simulink model "QPSK_BladeRF_tx"  (R2023a)
settings: Solver=FixedStepDiscrete  StartTime=0.0  StopTime=inf  RelTol=1e-3
undefined symbols (not defined in the file or in its folder): sdrqpsktx
libraries: dspsigops x2, commsequence2 x2, dspsrcs4 x2, commdigbbndpm3 x2, commfilt2 x2
settings Model: SimulationMode=accelerator  Creator=memre  LastModifiedBy=memre
settings DebuggingCC: ParameterPrecisionLossMsg=none
settings HardwareCC: ProdBitPerLong=64  ProdHWDeviceType=Intel->x86-64 (Linux 64)
settings RTWCC: Description=Simulink Desktop Real-Time  SystemTargetFile=sldrt.tlc  TemplateMakefile=sldrt.tmf  RTWCompilerOptimization=on
settings CodeAppCC: MaxIdLength=95
settings SimulinkDesktopRealTimeCC: TargetLibSuffix=_sldrt.a  TargetPreCompLibLocation=C:\Program Files\MATLAB\R2023a\toolbox\sldrt\lib\win64

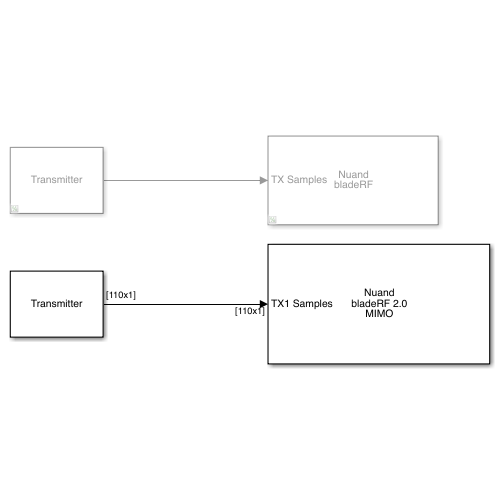
[thumbnail: Simulink's stored preview of the top-level diagram]
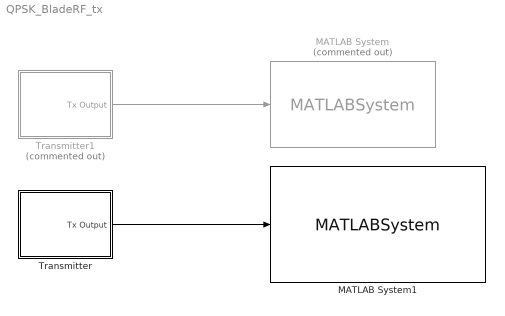
== system QPSK_BladeRF_tx ==
  MATLAB System : MATLABSystem  Commented=on  System=bladeRF_Simulink  device_string=*:instance=1  loopback_mode=None  xb200=off  SimulateUsing=Interpreted execution  enable_rx=off  enable_overrun=off  rx_frequency=sdrqpsktx.BladeRF_Frequency  rx_samplerate=sdrqpsktx.BladeRF_SampleRate  rx_bandwidth=1.5  rx_gain=sdrqpsktx.BladeRF_Gain_Rx  enable_rx_biastee=off  rx_agc=SLOW  rx_num_buffers=sdrqpsktx.BladeRF.stream.n_buffers  rx_num_transfers=sdrqpsktx.BladeRF.stream.n_transfers  rx_buf_size=sdrqpsktx.BladeRF.stream.buffer_size  rx_timeout_ms=sdrqpsktx.BladeRF.stream.timeout  rx_step_size=sdrqpsktx.BladeRF_FrameLength  enable_tx=on  enable_underrun=off  tx_frequency=sdrqpsktx.BladeRF_Frequency  tx_samplerate=sdrqpsktx.BladeRF_SampleRate  tx_bandwidth=1.5  tx_gain=sdrqpsktx.BladeRF_Gain_Tx  enable_tx_biastee=off  tx_num_buffers=sdrqpsktx.BladeRF.stream.n_buffers  tx_num_transfers=sdrqpsktx.BladeRF.stream.n_transfers  tx_buf_size=sdrqpsktx.BladeRF.stream.buffer_size  tx_timeout_ms=sdrqpsktx.BladeRF.stream.timeout  tx_step_size=sdrqpsktx.BladeRF_FrameLength  verbosity=Info
      mask Type: bladeRF_Simulink
      mask Display:
      | disp(['Nuand' char(10) 'bladeRF']);
      | port_label('input',1,'TX Samples');
  MATLAB System1 : MATLABSystem  System=bladeRF_MIMO_Simulink  device_string=*:instance=1  loopback_mode=None  xb200=off  SimulateUsing=Interpreted execution  enable_rx=off  enable_overrun=off  rx_frequency=sdrqpsktx.BladeRF_Frequency  rx_samplerate=sdrqpsktx.BladeRF_SampleRate  rx_bandwidth=1.5  rx_gain=sdrqpsktx.BladeRF_Gain_Rx  enable_rx_biastee=off  rx_agc=SLOW  rx_num_buffers=sdrqpsktx.BladeRF.stream.n_buffers  rx_num_transfers=sdrqpsktx.BladeRF.stream.n_transfers  rx_buf_size=sdrqpsktx.BladeRF.stream.buffer_size  rx_timeout_ms=sdrqpsktx.BladeRF.stream.timeout  rx_step_size=sdrqpsktx.BladeRF_FrameLength  enable_rx2=off  rx2_frequency=sdrqpsktx.BladeRF_Frequency  rx2_samplerate=sdrqpsktx.BladeRF_SampleRate  rx2_bandwidth=1.5  rx2_gain=sdrqpsktx.BladeRF_Gain_Rx  enable_rx2_biastee=off  rx2_agc=SLOW  enable_tx=on  enable_underrun=off  tx_frequency=sdrqpsktx.BladeRF_Frequency  tx_samplerate=sdrqpsktx.BladeRF_SampleRate  tx_bandwidth=1.5  tx_gain=sdrqpsktx.BladeRF_Gain_Tx  enable_tx_biastee=off  tx_num_buffers=sdrqpsktx.BladeRF.stream.n_buffers  tx_num_transfers=sdrqpsktx.BladeRF.stream.n_transfers  tx_buf_size=sdrqpsktx.BladeRF.stream.buffer_size  tx_timeout_ms=sdrqpsktx.BladeRF.stream.timeout  tx_step_size=sdrqpsktx.BladeRF_FrameLength  enable_tx2=off  tx2_frequency=sdrqpsktx.BladeRF_Frequency  tx2_samplerate=sdrqpsktx.BladeRF_SampleRate  tx2_bandwidth=1.5  tx2_gain=sdrqpsktx.BladeRF_Gain_Tx  enable_tx2_biastee=off  verbosity=Info
      mask Type: bladeRF_MIMO_Simulink
      mask Display:
      | disp(['Nuand' char(10) 'bladeRF 2.0' char(10) 'MIMO']);
      | port_label('input',1,'TX1 Samples');
  Transmitter : Subsystem
      mask Display: disp('Transmitter')
  Transmitter1 : Subsystem  Commented=on
      mask Display: disp('Transmitter')
  wires:
  Transmitter/1(Tx Output) -> MATLAB System1/1
  Transmitter1/1(Tx Output) -> MATLAB System/1

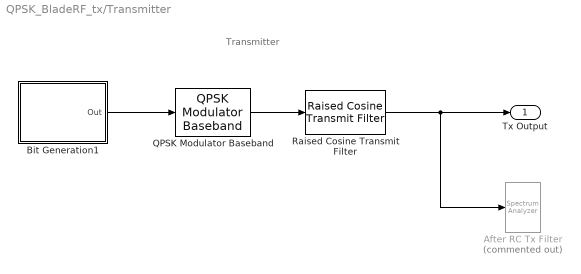
== system QPSK_BladeRF_tx/Transmitter ==
  note: Transmitter
  After RC Tx Filter : SpectrumAnalyzer  Commented=on  ScopeFrameLocation=window  Method=Welch  SampleRate=200000  Span=200000  StartFrequency=-100000  StopFrequency=100000  RBWSource=Property  RBW=750  FFTLength=128  AveragingMethod=Running  SpectralAverages=2  SpectrumUnits=dBW  YLabel=Spectrum after Raised-Cosine Tx Filter  YLimits=[-114.15736879359562 -6.4493918406395565]
      settings: OpenAtSimulationStart=off
  Bit Generation1 : Subsystem
      mask Display: disp('Bits Generation')
  QPSK Modulator Baseband : commdigbbndpm3/QPSK Modulator Baseband  InType=Bit  Enc=Gray  Ph=pi/4  outDtype=double  outWordLen=16  outUDDataType=sfix(16)  outFracLenMode=Best precision  outFracLen=15  outDataTypeStr=double  outLastDataTypeStr=double
  Raised Cosine Transmit Filter : commfilt2/Raised Cosine Transmit Filter  filtType=Square root  R=sdrqpsktx.RolloffFactor  filtSpan=sdrqpsktx.RaisedCosineFilterSpan  N=sdrqpsktx.Interpolation  filterGain=1  InputProcessing=Columns as channels (frame based)  RateOptions=Enforce single-rate processing  framing=Mute  checkCoeff=off  variableName=rcTxFilt1  checkGain=Normalized  sampMode=Mute  saveAsFlag=0  currentFiltSpan=10  D=5  launchFVT=on  roundingMode=Floor  overflowMode=off  coeffDataTypeStr=Inherit: Same word length as input  coeffMin=[]  coeffMax=[]  coeffLastDataTypeStr=Inherit: Same word length as input  outputDataTypeStr=Inherit: Same as accumulator  outputMin=[]  outputMax=[]  outputLastDataTypeStr=Inherit: Same as accumulator
  Tx Output : Outport  VectorParamsAs1DForOutWhenUnconnected=off
  wires:
  QPSK Modulator Baseband/1 -> Raised Cosine Transmit Filter/1
  Raised Cosine Transmit Filter/1 -> Tx Output/1, After RC Tx Filter/1
  Bit Generation1/1(Out) -> QPSK Modulator Baseband/1

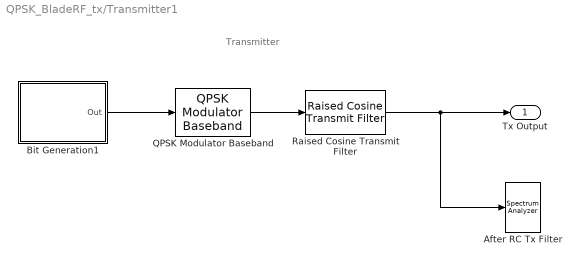
== system QPSK_BladeRF_tx/Transmitter1 ==
  note: Transmitter
  After RC Tx Filter : SpectrumAnalyzer  ScopeFrameLocation=window  Method=Welch  SampleRate=200000  Span=200000  StartFrequency=-100000  StopFrequency=100000  RBWSource=Property  RBW=750  FFTLength=128  AveragingMethod=Running  SpectralAverages=2  SpectrumUnits=dBW  YLabel=Spectrum after Raised-Cosine Tx Filter  YLimits=[-114.15736879359562 -6.4493918406395565]
      settings: OpenAtSimulationStart=off
  Bit Generation1 : Subsystem
      mask Display: disp('Bits Generation')
  QPSK Modulator Baseband : commdigbbndpm3/QPSK Modulator Baseband  InType=Bit  Enc=Gray  Ph=pi/4  outDtype=double  outWordLen=16  outUDDataType=sfix(16)  outFracLenMode=Best precision  outFracLen=15  outDataTypeStr=double  outLastDataTypeStr=double
  Raised Cosine Transmit Filter : commfilt2/Raised Cosine Transmit Filter  filtType=Square root  R=sdrqpsktx.RolloffFactor  filtSpan=sdrqpsktx.RaisedCosineFilterSpan  N=sdrqpsktx.Interpolation  filterGain=1  InputProcessing=Columns as channels (frame based)  RateOptions=Enforce single-rate processing  framing=Mute  checkCoeff=off  variableName=rcTxFilt1  checkGain=Normalized  sampMode=Mute  saveAsFlag=0  currentFiltSpan=10  D=5  launchFVT=on  roundingMode=Floor  overflowMode=off  coeffDataTypeStr=Inherit: Same word length as input  coeffMin=[]  coeffMax=[]  coeffLastDataTypeStr=Inherit: Same word length as input  outputDataTypeStr=Inherit: Same as accumulator  outputMin=[]  outputMax=[]  outputLastDataTypeStr=Inherit: Same as accumulator
  Tx Output : Outport  VectorParamsAs1DForOutWhenUnconnected=off
  wires:
  QPSK Modulator Baseband/1 -> Raised Cosine Transmit Filter/1
  Raised Cosine Transmit Filter/1 -> Tx Output/1, After RC Tx Filter/1
  Bit Generation1/1(Out) -> QPSK Modulator Baseband/1

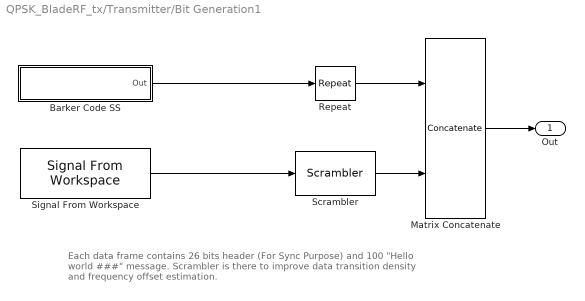
== system QPSK_BladeRF_tx/Transmitter/Bit Generation1 ==
  note: Each data frame contains 26 bits header (For Sync Purpose) and 100
      | "Hello world ###" message. Scrambler is there to improve data
      | transition density and frequency offset estimation.
  Barker Code SS : Subsystem
      mask Display: disp('Unipolar\nBarker Code')
  Matrix Concatenate : Concatenate  Mode=Multidimensional array
  Repeat : dspsigops/Repeat  FactorSource=Dialog parameter  N=2  Nmax=16  InputProcessing=Columns as channels (frame based)  RateOptions=Enforce single-rate processing  ic=0  mode=Unused parameter value
  Scrambler : commsequence2/Scrambler  M=2  poly=[1 1 1 0 1]  iniStaSource=Dialog Parameter  ini_sta=[0 0 0 0]  resetViaPort=off
  Signal From Workspace : dspsrcs4/Signal From Workspace  X=sdrqpsktx.MessageBits  Ts=1/sdrqpsktx.PayloadLength*sdrqpsktx.FrameTime  nsamps=sdrqpsktx.MessageLength * 7 * sdrqpsktx.NumberOfMessage  OutputAfterFinalValue=Cyclic repetition  ignoreOrWarnInputAndFrameLengths=off  OutputFrames=off
  Out : Outport  VectorParamsAs1DForOutWhenUnconnected=off
  wires:
  Barker Code SS/1(Out) -> Repeat/1
  Matrix Concatenate/1 -> Out/1
  Repeat/1 -> Matrix Concatenate/1
  Scrambler/1 -> Matrix Concatenate/2
  Signal From Workspace/1 -> Scrambler/1

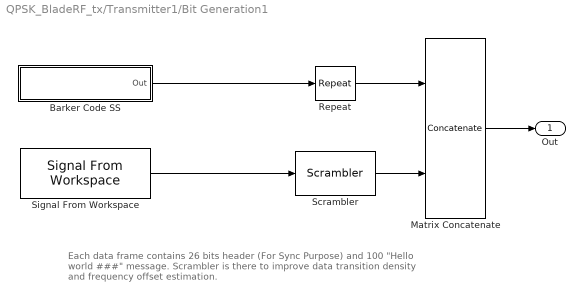
== system QPSK_BladeRF_tx/Transmitter1/Bit Generation1 ==
  note: Each data frame contains 26 bits header (For Sync Purpose) and 100
      | "Hello world ###" message. Scrambler is there to improve data
      | transition density and frequency offset estimation.
  Barker Code SS : Subsystem
      mask Display: disp('Unipolar\nBarker Code')
  Matrix Concatenate : Concatenate  Mode=Multidimensional array
  Repeat : dspsigops/Repeat  FactorSource=Dialog parameter  N=2  Nmax=16  InputProcessing=Columns as channels (frame based)  RateOptions=Enforce single-rate processing  ic=0  mode=Unused parameter value
  Scrambler : commsequence2/Scrambler  M=2  poly=[1 1 1 0 1]  iniStaSource=Dialog Parameter  ini_sta=[0 0 0 0]  resetViaPort=off
  Signal From Workspace : dspsrcs4/Signal From Workspace  X=sdrqpsktx.MessageBits  Ts=1/sdrqpsktx.PayloadLength*sdrqpsktx.FrameTime  nsamps=sdrqpsktx.MessageLength * 7 * sdrqpsktx.NumberOfMessage  OutputAfterFinalValue=Cyclic repetition  ignoreOrWarnInputAndFrameLengths=off  OutputFrames=off
  Out : Outport  VectorParamsAs1DForOutWhenUnconnected=off
  wires:
  Barker Code SS/1(Out) -> Repeat/1
  Matrix Concatenate/1 -> Out/1
  Repeat/1 -> Matrix Concatenate/1
  Scrambler/1 -> Matrix Concatenate/2
  Signal From Workspace/1 -> Scrambler/1

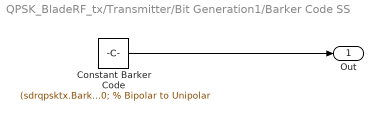
== system QPSK_BladeRF_tx/Transmitter/Bit Generation1/Barker Code SS ==
  Constant Barker Code : Constant  Value=(sdrqpsktx.BarkerCode)' > 0; % Bipolar to Unipolar  VectorParams1D=off  OutDataTypeStr=double
  Out : Outport  VectorParamsAs1DForOutWhenUnconnected=off
  wires:
  Constant Barker Code/1 -> Out/1

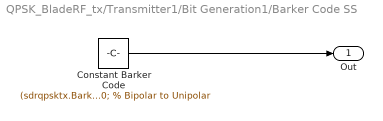
== system QPSK_BladeRF_tx/Transmitter1/Bit Generation1/Barker Code SS ==
  Constant Barker Code : Constant  Value=(sdrqpsktx.BarkerCode)' > 0; % Bipolar to Unipolar  VectorParams1D=off  OutDataTypeStr=double
  Out : Outport  VectorParamsAs1DForOutWhenUnconnected=off
  wires:
  Constant Barker Code/1 -> Out/1
